simulink library "PowerFlowLib"  (R2016a)
settings: Solver=ode45  StartTime=0.0  StopTime=10.0  RelTol=1e-3
undefined symbols (not defined in the file or in its folder): Air, AirProp, C, F1, F2, Fanmap, Fld1, Fld2, Fluid, fueltankdata, HydProp, HydraulicLoad, IBFD_exc, L, LoadFluidProps, magnitude, MSSN, n_alghts, PumpProp, pwr_alghts, R_fd_exc, Rcore, Ts, VBFD_exc
libraries: PowerFlowLib x35, simulink x19, powerlib_extras x2, dspstat3 x2
(part 8 of 12)

== system PowerFlowLib/Energy & Power Systems/Electrical/Systems/Generator Bus ==
  Select : Inport
  MAIN_Gen : Inport  Port=2
  APU_Gen : Inport  Port=3
  GND_sup : Inport  Port=4
  AUX_sup : Inport  Port=5
  i_Bus : Inport  Port=6
  Compare To Constant : Subsystem  mask(Compare To Constant){relop===, const=1, LogicOutDataTypeMode=uint8, ZeroCross=on}
      mask prompts: relop "Operator:"; const "Constant value:"; LogicOutDataTypeMode "Output data type mode:"; ZeroCross "Enable zero-crossing detection"
      mask help: Determine how a signal compares to a constant.
      mask init:
      | blkName = gcb;
      | 
      | if strcmp(get_param(gcbh,'LogicOutDataTypeMode'),'boolean')
      | 	setValue = 'Boolean';
      | else
      | 	setValue = 'Specify via dialog';
      | end
      | 
      | set_param([blkName,'/Compare'],'relop',relop, ...
      | 	'LogicOutDataTypeMode', setValue, 'ZeroCross', ZeroCross);
      | 
      | str = [relop,' C']; %default
      | 
      | const_str = get_param(blkName, 'const');
      | 
      | if isempty(strfind(const_str, ' ')) && isempty(strfind(const_str, ','))
      |     % scalar or single expression
      |     if isempty(str2num(const_str))
      |         %expression
      |         str = [relop, ' ', const_str];
      |     elseif length(const) == 1
      |         str = [relop,' ',num2str(double(const))];
      |     end
      | end
      mask TypeOptions relop: == | ~= | < | <= | >= | >
      mask TypeOptions LogicOutDataTypeMode: uint8 | boolean
      mask Callback ZeroCross: sl('zeroCrossEnable', gcbh);
      mask Display: disp(str)
  Compare To Constant1 : Subsystem  mask(Compare To Constant){relop===, const=2, LogicOutDataTypeMode=uint8, ZeroCross=on}
      mask prompts: relop "Operator:"; const "Constant value:"; LogicOutDataTypeMode "Output data type mode:"; ZeroCross "Enable zero-crossing detection"
      mask help: Determine how a signal compares to a constant.
      mask init: same as PowerFlowLib/Energy & Power Systems/Electrical/Systems/Generator Bus/Compare To Constant
      mask TypeOptions relop: == | ~= | < | <= | >= | >
      mask TypeOptions LogicOutDataTypeMode: uint8 | boolean
      mask Callback ZeroCross: sl('zeroCrossEnable', gcbh);
      mask Display: disp(str)
  Compare To Constant2 : Subsystem  mask(Compare To Constant){relop===, const=3, LogicOutDataTypeMode=uint8, ZeroCross=on}
      mask prompts: relop "Operator:"; const "Constant value:"; LogicOutDataTypeMode "Output data type mode:"; ZeroCross "Enable zero-crossing detection"
      mask help: Determine how a signal compares to a constant.
      mask init: same as PowerFlowLib/Energy & Power Systems/Electrical/Systems/Generator Bus/Compare To Constant
      mask TypeOptions relop: == | ~= | < | <= | >= | >
      mask TypeOptions LogicOutDataTypeMode: uint8 | boolean
      mask Callback ZeroCross: sl('zeroCrossEnable', gcbh);
      mask Display: disp(str)
  Compare To Constant3 : Subsystem  mask(Compare To Constant){relop===, const=4, LogicOutDataTypeMode=uint8, ZeroCross=on}
      mask prompts: relop "Operator:"; const "Constant value:"; LogicOutDataTypeMode "Output data type mode:"; ZeroCross "Enable zero-crossing detection"
      mask help: Determine how a signal compares to a constant.
      mask init: same as PowerFlowLib/Energy & Power Systems/Electrical/Systems/Generator Bus/Compare To Constant
      mask TypeOptions relop: == | ~= | < | <= | >= | >
      mask TypeOptions LogicOutDataTypeMode: uint8 | boolean
      mask Callback ZeroCross: sl('zeroCrossEnable', gcbh);
      mask Display: disp(str)
  Constant : Constant  Value=[0 0 0]
  Multiport Switch : MultiPortSwitch  Inputs=4
  Switch{,1..3} (4 alike) : Switch  Criteria=u2 ~= 0  Threshold=0.5
  Vbus : Outport
  i_MAIN : Outport  Port=2
  i_APU : Outport  Port=3
  i_GND : Outport  Port=4
  i_AUX : Outport  Port=5
  wires:
  MAIN_Gen/1 -> Multiport Switch/2
  APU_Gen/1 -> Multiport Switch/3
  GND_sup/1 -> Multiport Switch/4
  AUX_sup/1 -> Multiport Switch/5
  Multiport Switch/1 -> Vbus/1
  Select/1 -> Multiport Switch/1, Compare To Constant/1(u), Compare To Constant1/1(u), Compare To Constant2/1(u), Compare To Constant3/1(u)
  Switch/1 -> i_MAIN/1
  Switch1/1 -> i_APU/1
  Switch2/1 -> i_GND/1
  Switch3/1 -> i_AUX/1
  i_Bus/1 -> Switch/1, Switch1/1, Switch2/1, Switch3/1
  Compare To Constant/1(y) -> Switch/2
  Compare To Constant1/1(y) -> Switch1/2
  Compare To Constant2/1(y) -> Switch2/2
  Compare To Constant3/1(y) -> Switch3/2
  Constant/1 -> Switch3/3, Switch2/3, Switch1/3, Switch/3

== system PowerFlowLib/Energy & Power Systems/Electrical/Systems/Inverter Phase Control ==
  Constant : Constant  Value=pi/120
  Constant5 : Constant  Value=[1 0 0]
  Demux : Demux  Outputs=3
  Mux : Mux  Inputs=3
  Scope : Scope  NumInputPorts=2
  Sum : Sum  Inputs=|++
  Trigonometric Function : Trigonometry  Operator=atan2
  Trigonometric Function1 : Trigonometry
  Trigonometric Function2 : Trigonometry  Operator=cos
  q : Outport
  wires:
  Demux/1 -> Trigonometric Function/1
  Demux/2 -> Trigonometric Function/2
  Trigonometric Function/1 -> Sum/1
  Constant/1 -> Sum/2
  Sum/1 -> Trigonometric Function1/1, Trigonometric Function2/1
  Trigonometric Function1/1 -> Mux/1
  Trigonometric Function2/1 -> Mux/2
  Demux/3 -> Mux/3
  Mux/1 -> q/1, Scope/1
  Constant5/1 -> Demux/1

== system PowerFlowLib/Energy & Power Systems/Electrical/Systems/Transformer-rectifier ==
  vqd0 : Inport
  VDC : Inport  Port=2
  Bus Creator : BusCreator  Inputs=2
  Constant : Constant  Value=0.5*pu
  Memory33 : Memory
  Transformer1 : PowerFlowLib/Energy & Power Systems/Electrical/Machines/Transformer  Rp=0.005  Rs=0.1  N1=400  N2=197
  data_sink : PowerFlowLib/Support Functions//Tools/data_sink
  rectifier1 : PowerFlowLib/Energy & Power Systems/Electrical/Converters/rectifier  L=1e-1
  iout : Outport
  iqd0 : Outport  Port=2
  wires:
  vqd0/1 -> Transformer1/1
  VDC/1 -> rectifier1/3
  Transformer1/1 -> rectifier1/1
  Constant/1 -> rectifier1/2
  Memory33/1 -> Transformer1/2
  rectifier1/2 -> Memory33/1
  Transformer1/2 -> iqd0/1
  rectifier1/1 -> iout/1, Bus Creator/1  "Rectified Current (A)"
  Bus Creator/1 -> data_sink/1

== system PowerFlowLib/Energy & Power Systems/Electrical/Systems/three-phase full-bridge inverter ==
  qabc : Inport
  VDC : Inport  Port=2
  iabc : Inport  Port=3
  Add : Sum  Inputs=+
  Product : Product  SaturateOnIntegerOverflow=on  InputSameDT=on  OutDataTypeStr=Inherit: Same as first input
  Product1 : Product  SaturateOnIntegerOverflow=on  InputSameDT=on  OutDataTypeStr=Inherit: Same as first input
  Product2 : Product  RndMeth=Zero
  Scope : Scope
  Sqrt : Sqrt  SaturateOnIntegerOverflow=on
  Sum1 : Sum  Inputs=+
  Three-Phase Full Bridge Inverter CONSTANT FREQUENCY1 : Subsystem  mask{Tr=4e-6, Tf=3e-6, Fsw=2000, VCEsat=1, Nsw=6}
      mask prompts: Tr "Rise time for switching (s)"; Tf "Fall time for switching (s)"; Fsw "PWM Frequency (Hz)"; VCEsat "VCE saturation volt (V)"; Nsw "No. switches in inverter"
  Vabc : Outport
  Idc : Outport  Port=2
  Ploss : Outport  Port=3
  wires:
  [VDC] -> Product/2
  VDC/1 -> [VDC]
  Product/1 -> Vabc/1
  iabc/1 -> Product1/1, Product2/2, Product2/1
  qabc/1 -> [qabc]
  [qabc] -> Product/1
  [qabc] -> Product1/2
  Product1/1 -> Sum1/1
  Sum1/1 -> Idc/1
  [VDC] -> Three-Phase Full Bridge Inverter CONSTANT FREQUENCY1/1(Vdc)
  Add/1 -> Sqrt/1
  Product2/1 -> Add/1
  Sqrt/1 -> Three-Phase Full Bridge Inverter CONSTANT FREQUENCY1/2(Inverter current)
  Three-Phase Full Bridge Inverter CONSTANT FREQUENCY1/1(Total Loss) -> Scope/1, Ploss/1

== system PowerFlowLib/Energy & Power Systems/Hydraulic/Hydraulic Load/Reset Timer ==
  Reset : Inport
  Clock1 : Clock
  Clock3 : Clock
  Memory : Memory
  Sum1 : Sum  Inputs=|+-  SaturateOnIntegerOverflow=on  InputSameDT=on  OutDataTypeStr=Inherit: Same as first input
  Switch2 : Switch  Threshold=1  RndMeth=Zero
  Count : Outport
  wires:
  Clock1/1 -> Sum1/1
  Clock3/1 -> Switch2/3
  Switch2/1 -> Sum1/2, Memory/1
  Sum1/1 -> Count/1
  Reset/1 -> Switch2/2
  Memory/1 -> Switch2/1

== system PowerFlowLib/Energy & Power Systems/Thermal/ECS/ACM ==
  Flow In : Inport
  "Flow In " : Inport  Port=2
  Third Stream Air : Inport  Port=3
  Bus Selector1 : BusSelector  OutputSignals=temp_K
  Compressor : Subsystem
  Expanding Turbine : Subsystem
  Mux : Mux  Inputs=3
  Power Turbine : Subsystem
  Primary Heat Exchanger : Subsystem  mask{fld1=Air, fld2=Air, Tw_init=34, C_wall=60000, flow_switch=Upstream, Tw0=50, Q0=80000, H1_0=1500, A1=2.8702, mdot1_0=3, Tin1_0=15, H2_0=1500, A2=0.10566, mdot2_0=0.91, Tin2_0=600}
      mask prompts: fld1 "Fluid Type 1"; fld2 "Fluid Type 2"; Tw_init "Initial Wall Temperature [°C]"; C_wall "Wall Heat Capacitance  [J/K]"; flow_switch "Mass Flow Rate Calculated:"; Tw0 "Wall Temperature [°C]"; Q0 "Heat Transfer Rate [W]"; H1_0 "Heat Transfer Coefficient [W/m²K]"; A1 "Heat Transfer Area [m²]"; mdot1_0 "Mass Flow Rate [kg/s]"; Tin1_0 "Fluid Inlet Temperature[°C]"; H2_0 "Heat Transfer Coefficient [W/m²K]"; A2 "Heat Transfer Area [m²]"; mdot2_0 "Mass Flow Rate [kg/s]"; Tin2_0 "Fluid Inlet Temperature[°C]"
      mask init:
      | load Fluids
      | eval(['F1 = Fluid.',get_param(gcb,'fld1'),';']);
      | eval(['F2 = Fluid.',get_param(gcb,'fld2'),';']);
      | 
      | area1 = -(mdot1_0*F1.cp/H1_0)*...
      |               log(1-Q0/(mdot1_0*F1.cp*abs(Tw0-Tin1_0)));
      | 
      | set_param(gcb,'A1',num2str(area1));          
      |           
      | area2 = -(mdot2_0*F2.cp/H2_0)*...
      |               log(1-Q0/(mdot2_0*F2.cp*abs(-Tw0+Tin2_0)));   
      |           
      | set_param(gcb,'A2',num2str(area2));
      mask TypeOptions fld1: Fuel | Water | Air
      mask TypeOptions fld2: Fuel | Water | Air
      mask TypeOptions flow_switch: Upstream | Downstream
      mask Display:
      | text(0.5,0.95,['{\bf ',fld1,'/',fld2,' HX}'],'TexMode','on','horizontalAlignment', 'center')
      | 
      | port_label('input',1,[fld1,' In'])
      | port_label('input',2,[fld2,' In'])
      | port_label('output',1,[fld1,' Out'])
      | port_label('output',2,[fld2,' Out'])
  Scope : Scope  NumInputPorts=3
  Shaft : Subsystem
  Signal Routing : Subsystem
  Terminator1 : Terminator
  Terminator2 : Terminator
  Terminator3 : Terminator
  W to HP2 : Gain  Gain=0.00134102209
  rad 2 rev : Gain  Gain=60/2/pi
  Flow Out : Outport
  RPM : Outport  Port=2
  wires:
  Mux/1 -> Shaft/1(Power In/Out [vector])
  Shaft/1(Angular Velocity [rad/s]) -> rad 2 rev/1, Expanding Turbine/2(omega_rad/s), Compressor/2(omega_rad/s)
  Compressor/2(Power [W]) -> Scope/1, Mux/1
  Expanding Turbine/1(Power [W]) -> Scope/2, Mux/2
  Power Turbine/1(Power [W]) -> W to HP2/1, Scope/3, Mux/3
  "Flow In "/1 -> Power Turbine/1(Flow In)
  Compressor/1("Flow Out ") -> Primary Heat Exchanger/1(In1)
  Expanding Turbine/2(Flow Out) -> Flow Out/1
  Signal Routing/1(Flow Out) -> Primary Heat Exchanger/2(In2)
  Power Turbine/2(Flow Out) -> Terminator1/1
  rad 2 rev/1 -> RPM/1
  Third Stream Air/1 -> Bus Selector1/1, Signal Routing/1(Flow In)
  Bus Selector1/1 -> Power Turbine/2(temp_3rd)  "<temp_K>"
  Flow In/1 -> Compressor/1(Flow In)
  Primary Heat Exchanger/1(Out1) -> Expanding Turbine/1(Flow In)
  Primary Heat Exchanger/2(Out2) -> Terminator2/1
  W to HP2/1 -> Terminator3/1

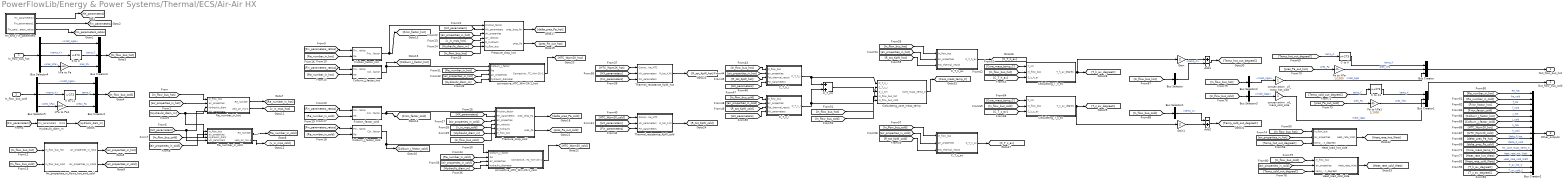
== system PowerFlowLib/Energy & Power Systems/Thermal/ECS/Air-Air HX ==
  In_flow_bus_hot : Inport
  In_flow_bus_cold : Inport  Port=2
  Add1 : Sum  Inputs=+-
  Add2 : Sum  Inputs=-+
  Air_properties_in_flows_hot_and_cold : Subsystem
  Bus Creator{,1,3..4} (4 alike) : BusCreator  Inputs=3
  Bus Creator2 : BusCreator  Inputs=15
  Bus Selector : BusSelector  OutputSignals=temp_C
  Bus Selector1 : BusSelector  OutputSignals=temp_C
  Bus Selector2 : BusSelector  OutputSignals=mdot_kgps
  Bus Selector3 : BusSelector  OutputSignals=mdot_kgps
  Bus Selector4 : BusSelector  OutputSignals=mdot_kgps,temp_K,pres_kPa
  Bus Selector5 : BusSelector  OutputSignals=mdot_kgps,temp_K,pres_kPa
  C to K : Bias  Bias=273
  C to K1 : Bias  Bias=273
  C_T_c_av : Subsystem
  C_T_c_i : Subsystem
  C_T_cm : Sum
  C_T_h_av : Subsystem
  C_T_h_i : Subsystem
  Calculating_T_c_av : Subsystem
  Calculating_T_h_av : Subsystem
  Calculating_core_mass_temp : Subsystem
  Colburn_J_factor_cold : Subsystem
  Colburn_J_factor_hot : Subsystem
  Friction_factor_cold : Subsystem
  Friction_factor_hot : Subsystem
  Gain : Gain  Gain=2
  Gain1 : Gain  Gain=2
  HX_and_Fin_paramters : Subsystem
  Heat_load_cold_side : Subsystem
  Heat_load_hot_side : Subsystem
  Hydraulic_diam_m : Subsystem
  K to C : Bias  Bias=-273
  K to C1 : Bias  Bias=-273
  Pa to kPa : Gain  Gain=1/1000
  Pa to kPa1 : Gain  Gain=1/1000
  Pressure_drop_cold : Subsystem
  Pressure_drop_hot : Subsystem
  Re_number_in_cold : Subsystem
  Re_number_in_hot : Subsystem
  Thermal_resistance_KpW_cold : Subsystem
  Thermal_resistance_KpW_hot : Subsystem
  conservation _of_mass_cold_side : Gain
  conservation _of_mass_hot_side : Gain
  convective_HTC_Wm-2K-1_cold : Subsystem
  convective_HTC_Wm-2K-1_hot : Subsystem
  kPa to Pa : Gain  Gain=1000
  kPa to Pa1 : Gain  Gain=1000
  Out_flow_bus_hot : Outport
  Out_flow_bus_cold : Outport  Port=2
  Other_outputs : Outport  Port=3
  wires:
  Heat_load_cold_side/1(Heat_rate_Watt) -> [Heat_rate_cold_Watt]
  [air_properties_in_cold] -> Heat_load_cold_side/2(air_properties)
  [In_flow_bus_cold] -> Heat_load_cold_side/1(In_flow_bus)
  [Temp_cold_out_degreeC] -> Heat_load_cold_side/3(temp_out_degreeC)
  Heat_load_hot_side/1(Heat_rate_Watt) -> [Heat_rate_hot_Watt]
  [air_properties_in_hot] -> Heat_load_hot_side/2(air_properties)
  [In_flow_bus_hot] -> Heat_load_hot_side/1(In_flow_bus)
  [Temp_hot_out_degreeC] -> Heat_load_hot_side/3(temp_out_degreeC)
  [R_tot_KpW_cold] -> C_T_c_av/3(Tot_thermal_resist)
  [air_properties_in_cold] -> C_T_c_av/2(air_properties)
  [In_flow_bus_cold] -> C_T_c_av/1(In_flow_bus)
  C_T_c_av/1(C_T_c_av) -> [C_T_c_av]
  Re_number_in_cold/2(velo_air_ms-1) -> [v_in_mps_cold]
  Bus Creator2/1 -> Other_outputs/1
  Bus Creator1/1 -> Out_flow_bus_cold/1
  Bus Creator/1 -> Out_flow_bus_hot/1
  conservation _of_mass_cold_side/1 -> Bus Creator1/3  "mdot_kgps"
  Bus Selector3/1 -> conservation _of_mass_cold_side/1  "<mdot_kgps>"
  conservation _of_mass_hot_side/1 -> Bus Creator/3  "mdot_kgps"
  Bus Selector2/1 -> conservation _of_mass_hot_side/1  "<mdot_kgps>"
  [In_flow_bus_cold] -> Bus Selector3/1
  [In_flow_bus_hot] -> Bus Selector2/1
  [pres_Pa_out_cold] -> Pa to kPa1/1  "pres_Pa"
  [Temp_cold_out_degreeC] -> C to K1/1  "temp_C"
  [pres_Pa_out_hot] -> Pa to kPa/1  "pres_Pa"
  [Temp_hot_out_degreeC] -> C to K/1  "temp_C"
  Add2/1 -> [Temp_cold_out_degreeC]
  Add1/1 -> [Temp_hot_out_degreeC]
  Bus Selector1/1 -> Add2/1  "<temp_C>"
  Gain1/1 -> Add2/2
  Bus Selector/1 -> Add1/2  "<temp_C>"
  Gain/1 -> Add1/1
  [In_flow_bus_cold] -> Bus Selector1/1
  [In_flow_bus_hot] -> Bus Selector/1
  Calculating_T_h_av/1(T_h_av_degreC) -> Gain/1, [T_h_av_degreeC]
  Calculating_T_c_av/1(T_c_av_degreC) -> Gain1/1, [T_c_av_degreeC]
  [C_T_c_av] -> Calculating_T_c_av/3(C_t_c_av)
  [In_flow_bus_cold] -> Calculating_T_c_av/2(In_flow_bus)
  [Core_mass_temp_C] -> Calculating_T_c_av/1(T_cm)
  [C_T_h_av] -> Calculating_T_h_av/3(C_t_h_av)
  C_T_h_av/1(C_T_h_av) -> [C_T_h_av]
  [In_flow_bus_hot] -> Calculating_T_h_av/2(In_flow_bus)
  [Core_mass_temp_C] -> Calculating_T_h_av/1(T_cm)
  Calculating_core_mass_temp/1(Core_mass_temp_C) -> [Core_mass_temp_C]
  [R_tot_KpW_hot] -> C_T_h_av/3(Tot_thermal_resist)
  [air_properties_in_hot] -> C_T_h_av/2(air_properties)
  [In_flow_bus_hot] -> C_T_h_av/1(In_flow_bus)
  [In_flow_bus_cold] -> Calculating_core_mass_temp/5(In_flow_bus_cold)
  [In_flow_bus_hot] -> Calculating_core_mass_temp/4(In_flow_bus_hot)
  C_T_cm/1 -> Calculating_core_mass_temp/3(C_t_cm)
  C_T_c_i/1(C_T_c_i) -> Calculating_core_mass_temp/2(C_T_c_i), C_T_cm/2
  C_T_h_i/1(C_T_h_i) -> Calculating_core_mass_temp/1(C_T_h_i), C_T_cm/1
  [HX_parameters] -> C_T_c_i/4(HX_parameters)
  [R_tot_KpW_cold] -> C_T_c_i/3(Tot_thermal_resist)
  [air_properties_in_cold] -> C_T_c_i/2(air_properties)
  [In_flow_bus_cold] -> C_T_c_i/1(In_flow_bus)
  [HX_parameters] -> C_T_h_i/4(HX_parameters)
  [R_tot_KpW_hot] -> C_T_h_i/3(Tot_thermal_resist)
  Thermal_resistance_KpW_cold/1(R_tot_K/W) -> [R_tot_KpW_cold]
  Thermal_resistance_KpW_hot/1(R_tot_K/W) -> [R_tot_KpW_hot]
  [air_properties_in_hot] -> C_T_h_i/2(air_properties)
  [In_flow_bus_hot] -> C_T_h_i/1(In_flow_bus)
  [HX_parameters] -> Thermal_resistance_KpW_cold/2(HX_parameters)
  [Fin_parameters] -> Thermal_resistance_KpW_cold/3(Fin_parameters)
  [HTC_Wpm2K_cold] -> Thermal_resistance_KpW_cold/1(Convective_HTC)
  [HX_parameters] -> Thermal_resistance_KpW_hot/2(HX_parameters)
  [Fin_parameters] -> Thermal_resistance_KpW_hot/3(Fin_parameters)
  [HTC_Wpm2K_hot] -> Thermal_resistance_KpW_hot/1(Convective_HTC)
  convective_HTC_Wm-2K-1_cold/1(Convective_HTC_Wm-2K-1) -> [HTC_Wpm2K_cold]
  convective_HTC_Wm-2K-1_hot/1(Convective_HTC_Wm-2K-1) -> [HTC_Wpm2K_hot]
  Pressure_drop_cold/2(pres_Pa) -> [pres_Pa_out_cold]
  Pressure_drop_hot/2(pres_Pa) -> [pres_Pa_out_hot]
  Pressure_drop_cold/1(pres_drop_Pa) -> [delta_pres_Pa_cold]
  Pressure_drop_hot/1(pres_drop_Pa) -> [delta_pres_Pa_hot]
  Colburn_J_factor_cold/1(Colburn_J_factor) -> convective_HTC_Wm-2K-1_cold/1(Colburn_J_factor), [Colburn_J_factor_cold]
  [Hydraulic_diam_m] -> convective_HTC_Wm-2K-1_cold/4(hydraulic_diameter)
  [air_properties_in_cold] -> convective_HTC_Wm-2K-1_cold/3(air_properties)
  [Re_number_in_cold] -> convective_HTC_Wm-2K-1_cold/2(Re)
  [Hydraulic_diam_m] -> convective_HTC_Wm-2K-1_hot/4(hydraulic_diameter)
  [air_properties_in_hot] -> convective_HTC_Wm-2K-1_hot/3(air_properties)
  [Re_number_in_hot] -> convective_HTC_Wm-2K-1_hot/2(Re)
  Colburn_J_factor_hot/1(Colburn_J_factor) -> convective_HTC_Wm-2K-1_hot/1(Colburn_J_factor), [Colburn_J_factor_hot]
  Friction_factor_cold/1(Friction_factor) -> Pressure_drop_cold/1(Friction_factor), [Fricn_factor_cold]
  [In_flow_bus_cold] -> Pressure_drop_cold/6(In_flow_bus)
  [Hydraulic_diam_m] -> Pressure_drop_cold/5(D_hydraulic)
  [v_in_mps_cold] -> Pressure_drop_cold/4(air_velocity)
  [air_properties_in_cold] -> Pressure_drop_cold/3(air_properties)
  [HX_parameters] -> Pressure_drop_cold/2(HX_parameters)
  [In_flow_bus_hot] -> Pressure_drop_hot/6(In_flow_bus)
  Friction_factor_hot/1(Friction_factor) -> Pressure_drop_hot/1(Friction_factor), [Fricn_factor_hot]
  [Hydraulic_diam_m] -> Pressure_drop_hot/5(D_hydraulic)
  [v_in_mps_hot] -> Pressure_drop_hot/4(air_velocity)
  [air_properties_in_hot] -> Pressure_drop_hot/3(air_properties)
  [HX_parameters] -> Pressure_drop_hot/2(HX_parameters)
  Re_number_in_hot/2(velo_air_ms-1) -> [v_in_mps_hot]
  [Re_number_in_cold] -> Colburn_J_factor_cold/2(Re)
  [Fin_parameters_ratios] -> Colburn_J_factor_cold/1(Fin_prameter_ratios)
  [Re_number_in_cold] -> Friction_factor_cold/2(Re)
  [Fin_parameters_ratios] -> Friction_factor_cold/1(Fin_prameter_ratios)
  [Re_number_in_hot] -> Colburn_J_factor_hot/2(Re)
  [Fin_parameters_ratios] -> Colburn_J_factor_hot/1(Fin_prameter_ratios)
  [Re_number_in_hot] -> Friction_factor_hot/2(Re)
  [Fin_parameters_ratios] -> Friction_factor_hot/1(Fin_prameter_ratios)
  HX_and_Fin_paramters/3(Fin_parameters_ratios) -> [Fin_parameters_ratios]
  [air_properties_in_cold] -> Re_number_in_cold/2(air_properties)
  [In_flow_bus_cold] -> Re_number_in_cold/1(In_flow_bus)
  [HX_parameters] -> Re_number_in_cold/4(HX_paramters), Re_number_in_hot/4(HX_paramters)
  [Hydraulic_diam_m] -> Re_number_in_cold/3(Hydraulic_diam), Re_number_in_hot/3(Hydraulic_diam)
  [air_properties_in_hot] -> Re_number_in_hot/2(air_properties)
  [In_flow_bus_hot] -> Re_number_in_hot/1(In_flow_bus)
  [In_flow_bus_cold] -> Air_properties_in_flows_hot_and_cold/2(In_flow_bus_cold)
  [In_flow_bus_hot] -> Air_properties_in_flows_hot_and_cold/1(In_flow_bus_hot)
  Air_properties_in_flows_hot_and_cold/2(air_properties_in_cold1) -> [air_properties_in_cold]
  Air_properties_in_flows_hot_and_cold/1(air_properties_in_hot1) -> [air_properties_in_hot]
  HX_and_Fin_paramters/2(Fin_parameters1) -> [Fin_parameters]
  HX_and_Fin_paramters/1(HX_parameters2) -> [HX_parameters]
  Re_number_in_cold/1(Re_number) -> [Re_number_in_cold]
  Re_number_in_hot/1(Re_number) -> [Re_number_in_hot]
  Hydraulic_diam_m/1(Out1) -> [Hydraulic_diam_m]
  [Fin_parameters] -> Hydraulic_diam_m/1(Fin_parameters)
  C to K/1 -> Bus Creator/1  "temp_K"
  Pa to kPa/1 -> Bus Creator/2  "pres_kPa"
  C to K1/1 -> Bus Creator1/1  "temp_K"
  Pa to kPa1/1 -> Bus Creator1/2  "pres_kPa"
  [Heat_rate_cold_Watt] -> Bus Creator2/13  "Heat_rate_cold_Watt"
  [Heat_rate_hot_Watt] -> Bus Creator2/12  "Heat_rate_hot_Watt"
  [Core_mass_temp_C] -> Bus Creator2/11  "HX_core_mass_temp_C"
  [Fricn_factor_hot] -> Bus Creator2/3  "f_hot"
  [Fricn_factor_cold] -> Bus Creator2/4  "f_cold"
  [Colburn_J_factor_hot] -> Bus Creator2/5  "J_hot"
  [Colburn_J_factor_cold] -> Bus Creator2/6  "J_cold"
  [HTC_Wpm2K_hot] -> Bus Creator2/7  "h_hot"
  [HTC_Wpm2K_cold] -> Bus Creator2/8  "h_cold"
  [delta_pres_Pa_hot] -> Bus Creator2/9  "Delta_P_hot"
  [delta_pres_Pa_cold] -> Bus Creator2/10  "Delta_P_cold"
  [Re_number_in_hot] -> Bus Creator2/1  "Re_hot"
  [Re_number_in_cold] -> Bus Creator2/2  "Re_cold"
  In_flow_bus_hot/1 -> Bus Selector4/1
  Bus Selector4/1 -> Bus Creator3/1  "<mdot_kgps>"
  Bus Selector4/2 -> K to C/1  "<temp_K>"
  Bus Selector4/3 -> kPa to Pa/1  "<pres_kPa>"
  K to C/1 -> Bus Creator3/2  "temp_C"
  Bus Creator3/1 -> [In_flow_bus_hot]
  kPa to Pa/1 -> Bus Creator3/3  "pres_Pa"
  Bus Selector5/1 -> Bus Creator4/1  "<mdot_kgps>"
  Bus Selector5/2 -> K to C1/1  "<temp_K>"
  Bus Selector5/3 -> kPa to Pa1/1  "<pres_kPa>"
  K to C1/1 -> Bus Creator4/2  "temp_C"
  kPa to Pa1/1 -> Bus Creator4/3  "press_Pa"
  Bus Creator4/1 -> [In_flow_bus_cold]
  [T_h_av_degreeC] -> Bus Creator2/14  "T_av_hot_C"
  [T_c_av_degreeC] -> Bus Creator2/15  "T_av_cold_C"
  In_flow_bus_cold/1 -> Bus Selector5/1

== system PowerFlowLib/Energy & Power Systems/Thermal/ECS/Cabin Zone ==
  note: Saturation added to
      | remove division by Zero
  Supply Air Flow In : Inport
  Amb Temp [K] : Inport  Port=2
  Mach_no : Inport  Port=3
  Thermal Load : Inport  Port=4
  Air Properties : Subsystem
  Bias : Bias  Bias=-273.15
  Bus Creator1 : BusCreator  Inputs=4
  Bus Creator2 : BusCreator  Inputs=2
  Bus Creator3 : BusCreator  Inputs=3
  Bus Creator4 : BusCreator  Inputs=3
  Bus Selector1 : BusSelector  OutputSignals=Cp_ra
  Bus Selector2 : BusSelector  OutputSignals=temp_K,mdot_kgps
  Bus Selector3 : BusSelector  OutputSignals=m_dot_ra
  C to K : Bias  Bias=273.15
  C to K1 : Bias  Bias=273.15
  Cabin Pressurization : Subsystem
  Cabin Temperature : Subsystem
  Cabin_parameters : Subsystem
  Gain : Gain
  Saturation : Saturate  UpperLimit=inf  LowerLimit=eps
  Terminator : Terminator
  calc_recirc_temp_ from_cab_temp : Sum
  data_sink : PowerFlowLib/Support Functions//Tools/data_sink
  m_dot_sa_required1 : Subsystem
  t_sa_term : Product  Inputs=*//
  Cabin Conditions : Outport
  Return Air  Conditions : Outport  Port=2
  wires:
  Saturation/1 -> t_sa_term/3
  calc_recirc_temp_ from_cab_temp/1 -> C to K1/1
  t_sa_term/1 -> calc_recirc_temp_ from_cab_temp/2
  [temp_cabin_C] -> calc_recirc_temp_ from_cab_temp/1
  Bus Selector3/1 -> Saturation/1, Gain/1  "<m_dot_ra>"
  Bus Selector1/1 -> t_sa_term/2  "<Cp_ra>"
  [Masses_cabin] -> Bus Selector3/1
  C to K1/1 -> Bus Creator3/1  "temp_K"
  Thermal Load/1 -> t_sa_term/1, Bus Creator4/3  "Thermal_Load"
  Mach_no/1 -> Cabin Temperature/6(Mach #)
  Amb Temp [K]/1 -> Cabin Temperature/5(Amb Temp [K])
  Supply Air Flow In/1 -> Bus Selector2/1, Air Properties/1(Supply Air)
  [temp_cabin_C] -> Cabin Pressurization/2(Cabin Temp. [C])
  Cabin Temperature/1(Cabin Temp. [C]) -> [temp_cabin_C], C to K/1  "temp_cabin_C"
  C to K/1 -> Bus Creator2/2, Bus Creator4/1  "temp_K"
  Bias/1 -> Cabin Temperature/1(Sup. Air Temp [C])
  m_dot_sa_required1/1(mdot SA Req.) -> Terminator/1
  Air Properties/3(Exhaust_AirProp) -> Bus Creator1/4
  Air Properties/2(Recirc_AirProp) -> Bus Selector1/1, Bus Creator1/3
  Air Properties/1(Supply_AirProp) -> m_dot_sa_required1/2(Sup. Air Prop.), Bus Creator1/2
  Bus Selector2/1 -> Bias/1  "<temp_K>"
  Air Properties/4(Cabin_AirProp) -> Cabin Pressurization/3(Cabin Prop.), Bus Creator1/1
  Cabin Pressurization/1(Cabin mdot & mass) -> [Masses_cabin], Cabin Temperature/2(Cabin mdot & mass)
  Cabin_parameters/1(Cabin Parameters) -> m_dot_sa_required1/1(Cabin Param.), Cabin Pressurization/4(Cabin Param.), Cabin Temperature/3(Cabin Param.)
  Bus Selector2/2 -> Cabin Pressurization/1(Sup. Air mdot)  "<mdot_kgps>"
  Bus Creator1/1 -> Cabin Temperature/4(Air Props.)
  Cabin Pressurization/2(Cabin Pres.) -> Bus Creator2/1, Bus Creator3/2, Bus Creator4/2  "pres_kPa"
  Bus Creator2/1 -> Cabin Conditions/1
  Bus Creator3/1 -> Return Air  Conditions/1
  Gain/1 -> Bus Creator3/3  "mdot_kgps"
  Bus Creator4/1 -> data_sink/1

== system PowerFlowLib/Energy & Power Systems/Thermal/ECS/Cargo bay ==
  note: Upper limit
      | to cargo temp.,
      | T_limit
  Return Air  Conditions : Inport
  "Thermal Loads, Q" : Inport  Port=2
  Flow from Right Pack : Inport  Port=3
  Add : Sum  Inputs=+++
  Add1 : Sum
  Bias : Bias  Bias=0.001
  Bus Creator : BusCreator  Inputs=3
  Bus Selector1 : BusSelector  OutputSignals=temp_K,mdot_kgps
  Bus Selector2 : BusSelector  OutputSignals=mdot_kgps,temp_K,pres_kPa
  Constant1 : Constant  Value=T_cargo_K
  Gain : Gain
  M_ra  x T_ra : Product
  M_right  x T_right : Product
  PID Controller1 : simulink/Continuous/PID Controller  Controller=PID  TimeDomain=Continuous-time  SampleTime=1  IntegratorMethod=Forward Euler  FilterMethod=Forward Euler  Form=Parallel  P=0.01  I=.01  D=0.01  N=100  InitialConditionSource=internal  InitialConditionForIntegrator=0  InitialConditionForFilter=0  ExternalReset=none  LimitOutput=on  UpperSaturationLimit=0.5  LowerSaturationLimit=.01  LinearizeAsGain=off  AntiWindupMode=none  Kb=1  TrackingMode=off  Kt=1  PParamMin=[]  PParamMax=[]  IParamMin=[]  IParamMax=[]  DParamMin=[]  DParamMax=[]  NParamMin=[]  NParamMax=[]  KbParamMin=[]  KbParamMax=[]  KtParamMin=[]  KtParamMax=[]  POutMin=[]  POutMax=[]  IOutMin=[]  IOutMax=[]  DOutMin=[]  DOutMax=[]  NOutMin=[]  NOutMax=[]  KbOutMin=[]  KbOutMax=[]  KtOutMin=[]  KtOutMax=[]  IntegratorOutMin=[]  IntegratorOutMax=[]  FilterOutMin=[]  FilterOutMax=[]  SumOutMin=[]  SumOutMax=[]  SumI1OutMin=[]  SumI1OutMax=[]  SumI2OutMin=[]  SumI2OutMax=[]  SumI3OutMin=[]  SumI3OutMax=[]  SumDOutMin=[]  SumDOutMax=[]  SaturationOutMin=[]  SaturationOutMax=[]  IntegratorContinuousStateAttributes=''  IntegratorStateMustResolveToSignalObject=off  IntegratorRTWStateStorageClass=Auto  FilterContinuousStateAttributes=''  FilterStateMustResolveToSignalObject=off  FilterRTWStateStorageClass=Auto
  Q/Cp : Product  Inputs=*/
  "Specific heat, Cp" : Constant  Value=1005
  Sum1 : Sum  Inputs=-+|
  T_out : Product  Inputs=*/
  data_sink : PowerFlowLib/Support Functions//Tools/data_sink
  Flow Distributor : Outport
  From cargo to fan : Outport  Port=2
  wires:
  Bias/1 -> Bus Creator/2, T_out/2  "mdot_kgps"
  M_ra  x T_ra/1 -> Add/3
  T_out/1 -> Sum1/2, Bus Creator/1  "temp_K"
  Bus Selector2/3 -> Gain/1  "<pres_kPa>"
  Bus Creator/1 -> data_sink/1, From cargo to fan/1
  Add/1 -> T_out/1
  Q/Cp/1 -> Add/2
  "Specific heat, Cp"/1 -> Q/Cp/2
  "Thermal Loads, Q"/1 -> Q/Cp/1
  Bus Selector2/2 -> M_ra  x T_ra/2  "<temp_K>"
  Bus Selector2/1 -> M_ra  x T_ra/1, Add1/2  "<mdot_kgps>"
  Add1/1 -> Bias/1  "mdot_kgps"
  M_right  x T_right/1 -> Add/1
  Bus Selector1/2 -> M_right  x T_right/2, Add1/1  "<mdot_kgps>"
  Bus Selector1/1 -> M_right  x T_right/1  "<temp_K>"
  Flow from Right Pack/1 -> Bus Selector1/1
  Sum1/1 -> PID Controller1/1
  Return Air  Conditions/1 -> Bus Selector2/1
  Constant1/1 -> Sum1/1
  PID Controller1/1 -> Flow Distributor/1  "Increase flow rate from the right pack"
  Gain/1 -> Bus Creator/3  "pres_kPa"

== system PowerFlowLib/Energy & Power Systems/Thermal/ECS/Compressor ==
  note: eff
  note: N
  note: Flow
  In2 : Inport
  In4 : Inport  Port=2
  Add : Sum
  Bias : Bias  Bias=-1
  Bus Creator1 : BusCreator  Inputs=3
  Bus Selector : BusSelector  OutputSignals=pres_kPa
  Bus Selector1 : BusSelector  OutputSignals=mdot_kgps
  Bus Selector2 : BusSelector  OutputSignals=temp_K
  Cp(P,T)1 : Lookup_n-D  BreakpointsForDimension1=AirProp.P  BreakpointsForDimension2=AirProp.T  BreakpointsForDimension3=[1]  Table=AirProp.Cp_pt  RndMeth=Simplest  InputSameDT=on
  Divide1 : Product  Inputs=/**
  Divide2 : Product  Inputs=***
  Divide3 : Product  Inputs=**
  Divide4 : Product  Inputs=/*
  Divide5 : Product  Inputs=/**
  Gain1 : Gain  Gain=1000
  K to R : Gain  Gain=1.8
  Math Function : Math  Operator=pow  SaturateOnIntegerOverflow=on
  Pressure_ratio : Lookup_n-D  BreakpointsForDimension1=[20,25,30,35,40,45,50,55,60,65,70,75,80,85,90]  BreakpointsForDimension2=[1097,1316,1536,1756,1975,2195,2414]  Table=reshape([1.22,1.202,1.18,1.145,1.05,1,1,1,1,1,1,1,1,1,1,1.325,1.31,1.3,1.275,1.22,1.16,1,1,1,1,1,1,1,1,1,1.49,1.485,1.475,1.45,1.41,1.38,1.3,1.15,1,1,1,1,1,1,1,1.65,1.65,1.63,1.628,1.61,1.598,1.55,1.5,1.4,1.1,1,1,1,1,1,1.885,1.87,1.87,1.86,1.83,1.82,1.8,1.76,1.7,1.62,1.5,1,1,1,1,2.15,2.15,2.15,2.14,2.12,2.05,2.085,2.05,2.01,1.98,1.902,1.8,1,1,1,2.45,2.44,2.43,2.42,2.41,2.405,2.4,2.39,2.365,2.32,2.28,2.2,2.14,2.02,1.7],15,7)  RndMeth=Simplest  InputSameDT=on
  Reciprocal Sqrt : Sqrt  SaturateOnIntegerOverflow=on
  Table1 : Lookup_n-D  BreakpointsForDimension1=[20,25,30,35,40,45,50,55,60,65,70,75,80,85,90]  BreakpointsForDimension2=[1097,1316,1536,1756,1975,2195,2414]  Table=reshape([0.84396,0.83224,0.7928,0.70795,0.33,0.16,0.16,0.16,0.16,0.16,0.16,0.16,0.16,0.16,0.16,0.8265,0.8272,0.823,0.8075,0.709,0.5437,0.0850000000000002,0.0850000000000002,0.0850000000000002,0.0850000000000002,0.0850000000000002,0.0850000000000002,0.0850000000000002,0.0850000000000002,0.0850000000000002,0.6962,0.716699999999999,0.753,0.8086,0.8094,0.777,0.672,0.3705,0.0690000000000002,0.0690000000000002,0.0690000000000002,0.0690000000000002,0.0690000000000002,0.0690000000000002,0.0690000000000002,0.803,0.803,0.8122,0.81312,0.82042,0.822052,0.8045,0.755,0.654,0.192,0.0480000000000002,0.0480000000000002,0.0480000000000002,0.0480000000000002,0.0480000000000002,0.79155,0.8025,0.8025,0.806,0.81335,0.8144,0.8165,0.811,0.7775,0.7328,0.628,0.0080000000000004,0.0080000000000004,0.0080000000000004,0.0080000000000004,0.802,0.802,0.802,0.802,0.802,0.8112,0.80584,0.8112,0.81728,0.80648,0.77466,0.723,0.00180000000000019,0.00180000000000019,0.00180000000000019,0.81,0.81,0.81,0.81,0.81,0.81,0.81,0.81,0.81,0.81,0.8068,0.7888,0.766,0.72408,0.54796],15,7)  RndMeth=Simplest  InputSameDT=on
  "m and P " : Gain  Gain=900
  poly index : Constant  Value=(1.4-1)/1.4
  Out1 : Outport
  Power_out : Outport  Port=2
  wires:
  Table1/1 -> Divide1/1
  "m and P "/1 -> Table1/1, Pressure_ratio/1
  Divide5/1 -> "m and P "/1
  Divide4/1 -> Table1/2, Pressure_ratio/2
  In4/1 -> Divide4/2
  K to R/1 -> Reciprocal Sqrt/1
  Bus Creator1/1 -> Out1/1
  Add/1 -> Bus Creator1/3  "temp_K"
  Divide3/1 -> Bus Creator1/1, Cp(P,T)1/1  "pres_kPa"
  Bus Selector/1 -> Divide5/1, Divide3/1  "<pres_kPa>"
  Divide2/1 -> Power_out/1
  Divide1/1 -> Add/1, Divide2/3, Cp(P,T)1/2
  Bias/1 -> Divide1/2
  Math Function/1 -> Bias/1
  poly index/1 -> Math Function/2
  Pressure_ratio/1 -> Divide3/2, Math Function/1
  Bus Selector1/1 -> Divide5/2, Bus Creator1/2, Divide2/1  "<mdot_kgps>"
  Reciprocal Sqrt/1 -> Divide5/3, Divide4/1
  Bus Selector2/1 -> K to R/1, Add/2, Divide1/3  "<temp_K>"
  In2/1 -> Bus Selector2/1, Bus Selector1/1, Bus Selector/1
  Cp(P,T)1/1 -> Gain1/1
  Gain1/1 -> Divide2/2

== system PowerFlowLib/Energy & Power Systems/Thermal/ECS/Fan ==
  Flow In : Inport
  Air Properties : Subsystem
  Bias : Bias  Bias=-273
  Bias1 : Bias  Bias=273
  Bus Creator{2,4..6} (4 alike) : BusCreator  Inputs=3
  Bus Selector : BusSelector  OutputSignals=Rho_in_kgpm3
  Bus Selector1 : BusSelector  OutputSignals=mdot_kgps
  Bus Selector2 : BusSelector  OutputSignals=mdot_kgps,temp_C,press_Pa
  Bus Selector3 : BusSelector  OutputSignals=temp_K,pres_kPa,mdot_kgps
  Calculating_vol_flow_rate : Product  Inputs=*/
  Constant : Constant  Value=N_fan
  Gain : Gain  Gain=1000
  Gain1 : Gain  Gain=1/1000
  Gain2 : Gain
  Gain3 : Gain
  Gain4 : Gain  Gain=1/1000
  Performance_curves_1725 rpm : Subsystem  TreatAsAtomicUnit=on
  m3ps_to_cfm : Gain  Gain=2118.88
  Flow Out : Outport
  Fan Data : Outport  Port=2
  wires:
  Constant/1 -> [Fan_speed_rpm]
  Bus Selector3/1 -> Bias/1  "<temp_K>"
  Gain4/1 -> Bus Creator5/2  "power_kW"
  Performance_curves_1725 rpm/1(Power_required_W) -> Gain4/1  "power_W"
  [Fan_speed_rpm] -> Bus Creator5/1  "fan_speed_rpm"
  Performance_curves_1725 rpm/2(fan_efficiency) -> Bus Creator5/3  "fan_efficiency"
  Performance_curves_1725 rpm/5(mass_kgps) -> Bus Creator4/3
  Performance_curves_1725 rpm/4(Temp_out_C) -> Bus Creator4/2
  Performance_curves_1725 rpm/3(Pressure_out_Pa) -> Bus Creator4/1
  Bus Creator4/1 -> Bus Selector2/1
  Bus Creator6/1 -> Flow Out/1
  Bus Creator5/1 -> Fan Data/1
  Bus Selector2/3 -> Gain1/1  "<press_Pa>"
  Bus Selector2/2 -> Bias1/1  "<temp_C>"
  Bus Selector2/1 -> Gain3/1  "<mdot_kgps>"
  Bias1/1 -> Bus Creator6/2  "temp_K"
  Gain1/1 -> Bus Creator6/3  "pres_kPa"
  Gain3/1 -> Bus Creator6/1  "mdot_kgps"
  [FlowIn] -> Performance_curves_1725 rpm/2(in_flow_bus)
  [Vol_flow_rate] -> Performance_curves_1725 rpm/1(Vol_flow_rate_cfm_in)
  [AirProp] -> Performance_curves_1725 rpm/3(Air_properties_at_inlet)
  m3ps_to_cfm/1 -> [Vol_flow_rate]
  Calculating_vol_flow_rate/1 -> m3ps_to_cfm/1
  Bus Selector1/1 -> Calculating_vol_flow_rate/1  "<mdot_kgps>"
  [FlowIn] -> Bus Selector1/1
  Bus Selector/1 -> Calculating_vol_flow_rate/2  "<Rho_in_kgpm3>"
  Air Properties/1(AirProp) -> [AirProp], Bus Selector/1
  Bus Creator2/1 -> [FlowIn]
  Flow In/1 -> Air Properties/1(Flow In), Bus Selector3/1
  Bias/1 -> Bus Creator2/1  "temp_C"
  Gain/1 -> Bus Creator2/2  "pres_Pa"
  Gain2/1 -> Bus Creator2/3  "mdot_kgps"
  Bus Selector3/2 -> Gain/1  "<pres_kPa>"
  Bus Selector3/3 -> Gain2/1  "<mdot_kgps>"

== system PowerFlowLib/Energy & Power Systems/Thermal/ECS/T_35_valve ==
  In1 : Inport
  In2 : Inport  Port=2
  Bus Creator1 : BusCreator  Inputs=3
  Bus Creator2 : BusCreator  Inputs=3
  Bus Selector1 : BusSelector  OutputSignals=temp_K,mdot_kgps,pres_kPa
  Bus Selector3 : BusSelector  OutputSignals=temp_K,mdot_kgps,pres_kPa
  Constant2 : Constant  Value=0
  Memoy1 : Memory
  Scope : Scope
  Subtract2 : Sum  Inputs=+-
  Subtract3 : Sum  Inputs=+-
  Subtract4 : Sum  Inputs=+-
  Switch2 : Switch
  Switch3 : Switch
  T_35F : Constant  Value=T_35
  Terminator : Terminator
  delta_m =m_c*(T_35-Tt)/(Tc-Tt) : Product  Inputs=/**
  Out2 : Outport
  Out1 : Outport  Port=2
  wires:
  T_35F/1 -> Subtract2/1, Switch3/1
  Bus Selector3/1 -> Subtract3/2, Subtract2/2, Switch3/3  "<temp_K>"
  Subtract2/1 -> delta_m =m_c*(T_35-Tt)/(Tc-Tt)/3
  Bus Selector1/2 -> delta_m =m_c*(T_35-Tt)/(Tc-Tt)/2, Subtract4/1, Bus Creator2/2  "<mdot_kgps>"
  Bus Selector1/1 -> Subtract3/1, Bus Creator1/1  "<temp_K>"
  Subtract3/1 -> delta_m =m_c*(T_35-Tt)/(Tc-Tt)/1
  delta_m =m_c*(T_35-Tt)/(Tc-Tt)/1 -> Switch2/2, Switch2/1, Switch3/2  "delta_m"
  Constant2/1 -> Switch2/3
  Switch2/1 -> Memoy1/1
  Bus Selector1/3 -> Bus Creator1/2  "<pres_kPa>"
  Memoy1/1 -> Subtract4/2, Scope/1
  Subtract4/1 -> Bus Creator1/3  "mdot_kgps"
  Bus Creator1/1 -> Out1/1
  Switch3/1 -> Bus Creator2/1  "temp_K"
  Bus Selector3/3 -> Bus Creator2/3  "<pres_kPa>"
  Bus Selector3/2 -> Terminator/1  "<mdot_kgps>"
  Bus Creator2/1 -> Out2/1
  In1/1 -> Bus Selector1/1
  In2/1 -> Bus Selector3/1

== system PowerFlowLib/Energy & Power Systems/Thermal/ECS/Turbine ==
  note: Pt
  Flow : Inport
  W_compressor : Inport  Port=2
  Add : Sum  Inputs=+-
  Add1 : Sum  Inputs=-+
  Bias : Bias  Bias=-1
  Bus Creator : BusCreator  Inputs=3
  Bus Selector : BusSelector  OutputSignals=pres_kPa
  Bus Selector1 : BusSelector  OutputSignals=mdot_kgps
  Bus Selector2 : BusSelector  OutputSignals=temp_K
  Cp(P,T)1 : Lookup_n-D  BreakpointsForDimension1=AirProp.P  BreakpointsForDimension2=AirProp.T  BreakpointsForDimension3=[1]  Table=AirProp.Cp_pt  RndMeth=Simplest  InputSameDT=on
  Divide : Product  Inputs=/*
  Divide3 : Product  Inputs=***
  Divide4 : Product  Inputs=***
  Divide5 : Product  Inputs=/*
  Gain : Gain  Gain=-1
  Gain1 : Gain  Gain=1000
  Inertia : Constant  Value=inertia
  Integrator : Integrator  InitialCondition=1600000000
  Math Function : Math  Operator=pow  SaturateOnIntegerOverflow=on
  Reciprocal Sqrt : Sqrt  SaturateOnIntegerOverflow=on
  poly index : Constant  Value=(1.4-1)/1.4
  turbine efficiency : Constant  Value=n_t
  urbine Exit pressure : Constant  Value=press_Turbine_exit
  Flow_out : Outport
  N : Outport  Port=2
  W_turbine : Outport  Port=3
  wires:
  Bus Creator/1 -> Flow_out/1
  Gain/1 -> Divide3/2
  turbine efficiency/1 -> Divide3/3
  urbine Exit pressure/1 -> Divide/2, Bus Creator/3, Cp(P,T)1/2  "pres_kPa"
  Reciprocal Sqrt/1 -> N/1
  W_compressor/1 -> Add1/1
  Flow/1 -> Bus Selector2/1, Bus Selector1/1, Bus Selector/1
  Bus Selector/1 -> Divide/1  "<pres_kPa>"
  Divide/1 -> Math Function/1
  poly index/1 -> Math Function/2
  Math Function/1 -> Bias/1
  Bias/1 -> Gain/1
  Bus Selector2/1 -> Divide3/1, Add/1, Cp(P,T)1/1  "<temp_K>"
  Divide3/1 -> Divide4/3, Add/2
  Cp(P,T)1/1 -> Gain1/1
  Bus Selector1/1 -> Divide4/1, Bus Creator/1  "<mdot_kgps>"
  Divide4/1 -> W_turbine/1, Add1/2
  Add1/1 -> Divide5/2
  Inertia/1 -> Divide5/1
  Divide5/1 -> Integrator/1
  Integrator/1 -> Reciprocal Sqrt/1
  Add/1 -> Bus Creator/2  "temp_K"
  Gain1/1 -> Divide4/2

== system PowerFlowLib/Energy & Power Systems/Thermal/ECS/n-intlet Mixing Junction ==
  Inlet#1 : Inport
  Inlet#2 : Inport  Port=2
  Inlet#3 : Inport  Port=3
  Bias1 : Bias  Bias=-273
  Bias2 : Bias  Bias=273
  Bus Creator3 : BusCreator  Inputs=3
  BusSel#1 : BusSelector  OutputSignals=pres_kPa,temp_K,mdot_kgps
  BusSel#2 : BusSelector  OutputSignals=pres_kPa,temp_K,mdot_kgps
  BusSel#3 : BusSelector  OutputSignals=pres_kPa,temp_K,mdot_kgps
  Cp(P,T)2 : Lookup_n-D  BreakpointsForDimension1=AirProp.P  BreakpointsForDimension2=AirProp.T  BreakpointsForDimension3=[1]  Table=AirProp.Cp_pt  RndMeth=Simplest  InputSameDT=on
  Divide : Product  Inputs=***
  Divide1 : Product  Inputs=*/
  Divide2 : Product  Inputs=*/
  Divide3 : Product  Inputs=*//
  Gain1 : Gain  Gain=1000
  Sum of Elements{1..4} (4 alike) : Sum  Inputs=+
  Width : Width
  Width1 : Width
  mdot_vector : Concatenate  NumInputs=3
  pres_vector : Concatenate  NumInputs=3
  temp_vector : Concatenate  NumInputs=3
  Flow Out : Outport
  wires:
  Bias2/1 -> Bus Creator3/2  "temp_K"
  Bus Creator3/1 -> Flow Out/1
  temp_vector/1 -> Bias1/1  "temp_K"
  pres_vector/1 -> Cp(P,T)2/1, Sum of Elements4/1, Width1/1  "pres_kPa"
  Cp(P,T)2/1 -> Gain1/1  "Cp"
  mdot_vector/1 -> Sum of Elements1/1, Divide/3  "mdot"
  Sum of Elements1/1 -> Divide3/3, Bus Creator3/3  "mdot_kgps"
  Sum of Elements2/1 -> Divide2/1
  Width/1 -> Divide2/2
  Divide/1 -> Sum of Elements3/1
  Sum of Elements3/1 -> Divide3/1
  Divide2/1 -> Divide3/2
  Bias1/1 -> Divide/2, Cp(P,T)2/2
  Divide3/1 -> Bias2/1  "temp_C"
  Inlet#1/1 -> BusSel#1/1
  BusSel#1/1 -> pres_vector/1  "<pres_kPa>"
  BusSel#1/2 -> temp_vector/1  "<temp_K>"
  BusSel#1/3 -> mdot_vector/1  "<mdot_kgps>"
  Inlet#2/1 -> BusSel#2/1
  BusSel#2/1 -> pres_vector/2  "<pres_kPa>"
  BusSel#2/2 -> temp_vector/2  "<temp_K>"
  BusSel#2/3 -> mdot_vector/2  "<mdot_kgps>"
  Inlet#3/1 -> BusSel#3/1
  BusSel#3/1 -> pres_vector/3  "<pres_kPa>"
  BusSel#3/2 -> temp_vector/3  "<temp_K>"
  BusSel#3/3 -> mdot_vector/3  "<mdot_kgps>"
  Divide1/1 -> Bus Creator3/1  "pres_kPa"
  Sum of Elements4/1 -> Divide1/1
  Width1/1 -> Divide1/2
  Gain1/1 -> Sum of Elements2/1, Width/1, Divide/1

== system PowerFlowLib/Energy & Power Systems/Thermal/Fuel & Oil/Cold Plate ==
  Q : Inport
  In : Inport  Port=2
  Add : Sum  Inputs=+-
  Add1 : Sum  Inputs=-+
  Add2 : Sum
  Add3 : Sum  Inputs=-+
  Bias : Bias  Bias=eps
  Bus Creator : BusCreator  Inputs=3
  Bus Creator1 : BusCreator  Inputs=3
  Bus Selector : BusSelector  OutputSignals=mdot_kgps,temp_K,pres_kPa
  Cw : Constant  Value=C_wall
  Divide : Product  Inputs=*/
  Divide1 : Product  Inputs=**
  Divide2 : Product  Inputs=**
  Divide3 : Product  Inputs=**
  Divide4 : Product  Inputs=/**
  Gain : Gain  Gain=-1
  H_As1 : Constant  Value=4/5
  H_As4 : Constant  Value=(H0/mdot0^(4/5))*A
  Math Function : Math  SaturateOnIntegerOverflow=on
  Math Function3 : Math  Operator=pow  SaturateOnIntegerOverflow=on
  Tw : Integrator  InitialCondition=Tw_init
  cp : Constant  Value=Fluid.cp
  data_sink : PowerFlowLib/Support Functions//Tools/data_sink
  Out : Outport
  wires:
  Bias/1 -> Divide4/1
  Divide/1 -> Tw/1
  Cw/1 -> Divide/2
  Add/1 -> Divide/1
  cp/1 -> Divide1/1
  Add2/1 -> Bus Creator1/2, [T_out]  "T_out"
  Divide2/1 -> Add/2  "Q"
  Tw/1 -> Bus Creator1/1, Add2/1, Add3/1  "T_wall"
  Divide3/1 -> Add2/2
  Add3/1 -> Divide3/1
  Bus Creator/1 -> Out/1
  [m_dot] -> Bus Creator/1  "mdot_kgps"
  Q/1 -> [Q_Load]
  [Q_Load] -> Add/1
  Bus Selector/2 -> [T_in]  "<temp_K>"
  [T_in] -> Add1/1
  [T_out] -> Add1/2
  [T_out] -> Bus Creator/2  "temp_K"
  [T_in] -> Add3/2
  Math Function/1 -> Divide3/2
  Add1/1 -> Divide2/1
  Divide1/1 -> Divide2/2, Bias/1
  Divide4/1 -> Gain/1
  H_As4/1 -> Divide4/2
  Gain/1 -> Math Function/1
  Bus Selector/1 -> [m_dot]  "<mdot_kgps>"
  In/1 -> Bus Selector/1
  [m_dot] -> Math Function3/1, Divide1/2
  H_As1/1 -> Math Function3/2
  Math Function3/1 -> Divide4/3
  Bus Creator1/1 -> data_sink/1
  [Q_Load] -> Bus Creator1/3  "Q_load"
  Bus Selector/3 -> [pres_in]  "<pres_kPa>"
  [pres_in] -> Bus Creator/3  "pres_kPa"

== system PowerFlowLib/Energy & Power Systems/Thermal/Fuel & Oil/Flow Junction ==
  mdot Out : Inport
  Flow In 1 : Inport  Port=2
  Flow In 2 : Inport  Port=3
  Flow In 3 : Inport  Port=4
  Bus Creator : BusCreator  Inputs=4
  Bus Selector : BusSelector  OutputSignals=H_kJpkg
  Bus Selector1 : BusSelector  OutputSignals=H_kJpkg
  Bus Selector2 : BusSelector  OutputSignals=mdot_kgps
  Bus Selector3 : BusSelector  OutputSignals=mdot_kgps
  Bus Selector4 : BusSelector  OutputSignals=H_kJpkg
  Bus Selector5 : BusSelector  OutputSignals=mdot_kgps
  Integrator : Integrator  InitialCondition=initPres
  Integrator1 : Integrator  InitialCondition=interp2(F1.T,F1.P,F1.H_pt,initTemp,initPres)
  Liquid Enthalpy/Pressure Calcs : Subsystem
  Mux : Mux  Inputs=3
  Mux1 : Mux  Inputs=3
  T (p,h) : Lookup2D  RowIndex=F1.P  ColumnIndex=F1.H  Table=F1.T_ph  SaturateOnIntegerOverflow=on  InputSameDT=on
  Flow Out : Outport
  wires:
  Bus Selector5/1 -> Mux/3  "<mdot_kgps>"
  Flow In 3/1 -> Bus Selector5/1, Bus Selector4/1
  Bus Selector4/1 -> Mux1/3  "<H_kJpkg>"
  mdot Out/1 -> Bus Creator/4, Liquid Enthalpy/Pressure Calcs/1(Mdot_Out)  "mdot_kgps"
  Bus Creator/1 -> Flow Out/1  "Outlet"
  T (p,h)/1 -> Bus Creator/2  "temp_K"
  Flow In 1/1 -> Bus Selector/1, Bus Selector2/1  "Inlet1"
  Flow In 2/1 -> Bus Selector1/1, Bus Selector3/1  "Inlet2"
  [Pfluid] -> Liquid Enthalpy/Pressure Calcs/3(Pfluid)
  [Hfluid] -> Liquid Enthalpy/Pressure Calcs/2(Hfluid)
  Liquid Enthalpy/Pressure Calcs/2(Pdot) -> Integrator/1
  Integrator/1 -> [Pfluid], T (p,h)/1, Bus Creator/3  "pres_kPa"
  Mux/1 -> Liquid Enthalpy/Pressure Calcs/4(Mdot_In)
  Integrator1/1 -> [Hfluid], Bus Creator/1, T (p,h)/2  "H_kJpkg"
  Liquid Enthalpy/Pressure Calcs/1(Hdot) -> Integrator1/1
  Mux1/1 -> Liquid Enthalpy/Pressure Calcs/5(H_In)
  Bus Selector3/1 -> Mux/2  "<mdot_kgps>"
  Bus Selector2/1 -> Mux/1  "<mdot_kgps>"
  Bus Selector1/1 -> Mux1/2  "<H_kJpkg>"
  Bus Selector/1 -> Mux1/1  "<H_kJpkg>"

== system PowerFlowLib/Energy & Power Systems/Thermal/Fuel & Oil/Fluid Pump ==
  Flow_in : Inport
  w_rpm : Inport  Port=2
  P_out : Inport  Port=3
  (1-pf)/pf : Gain  Gain=(1-pf)/pf
  2- Lookup Table3 : Lookup_n-D  BreakpointsForDimension1=F1.P  BreakpointsForDimension2=F1.T  Table=F1.H_pt  RndMeth=Simplest  InputSameDT=on
  2pi : Gain  Gain=2*pi
  2pi/60 : Gain  Gain=2*pi()/60
  Add1 : Sum
  Add2 : Sum  Inputs=-+
  Add3 : Sum  Inputs=-+
  Bus Creator : BusCreator  Inputs=4
  Bus Creator1 : BusCreator  Inputs=3
  Bus Creator2 : BusCreator  Inputs=4
  Bus Selector : BusSelector  OutputSignals=temp_K,pres_kPa
  Constant1 : Constant  Value=pump_eff
  Cp (T,P) : Lookup_n-D  BreakpointsForDimension1=F1.P  BreakpointsForDimension2=F1.T  Table=F1.Cp_pt  RndMeth=Simplest  InputSameDT=on
  Demux : Demux  Outputs=2
  Divide2 : Product  Inputs=//*
  Divide3 : Product  Inputs=**
  Divide4 : Product  Inputs=**/
  Divide5 : Product  Inputs=**
  Divide7 : Product  Inputs=*/
  Multiport Switch : MultiPortSwitch
  Mux : Mux  Inputs=2
  Mux1 : Mux  Inputs=2
  Pump Vol. FlowRate : Lookup_n-D  NumberOfTableDimensions=1  BreakpointsForDimension1=PumpProp.B737_mech_fuel1.pres  Table=PumpProp.B737_mech_fuel1.q  RndMeth=Simplest  InputSameDT=on
  Switch : Switch  Criteria=u2 > Threshold
  Switch1 : Switch  Criteria=u2 > Threshold
  W to kW : Gain  Gain=1/1000
  data_sink : PowerFlowLib/Support Functions//Tools/data_sink
  heat_switch : Gain
  "kPa " : Gain
  kPa to Pa : Gain  Gain=1000
  kPa to bar : Gain  Gain=0.01
  kPa to m : Gain  Gain=.10197/SG
  kg/s : Gain  Gain=1/3600
  m^3/min : Gain  Gain=1/60
  pwr_switch : Constant  Value=0
  rho (T,P) : Lookup_n-D  BreakpointsForDimension1=F1.P  BreakpointsForDimension2=F1.T  Table=F1.Rho_pt  RndMeth=Simplest  InputSameDT=on
  switchcase : Constant  Value=2
  zero : Constant  Value=0
  zero1 : Constant  Value=0
  Flow_Out : Outport
  Pump Power : Outport  Port=2
  wires:
  kPa to bar/1 -> Multiport Switch/4
  "kPa "/1 -> Multiport Switch/3
  Multiport Switch/1 -> Pump Vol. FlowRate/1
  switchcase/1 -> Multiport Switch/1
  Divide4/1 -> Divide5/1  "Torq_Nm"
  Pump Vol. FlowRate/1 -> m^3/min/1, Divide3/2  "m^3/hr"
  Divide3/1 -> kg/s/1  "mdot_kgphr"
  kPa to m/1 -> Multiport Switch/2  "head (m)"
  [Pout] -> Add2/2
  [mdot] -> Bus Creator/2  "mdot_kgps"
  w_rpm/1 -> 2pi/1, 2pi/60/1, Bus Creator2/4, Switch/2, Switch/3  "shaftspeed_rpm"
  Add1/1 -> Bus Creator/3, 2- Lookup Table3/2  "temp_K"
  Add2/1 -> kPa to bar/1, "kPa "/1, kPa to m/1, kPa to Pa/1  "delta P"
  Bus Selector/2 -> Add2/1, Cp (T,P)/1, rho (T,P)/1  "<pres_kPa>"
  Bus Selector/1 -> Cp (T,P)/2, Add1/1, rho (T,P)/2  "<temp_K>"
  rho (T,P)/1 -> Divide3/1  "rho"
  Constant1/1 -> Divide7/2
  Cp (T,P)/1 -> Divide2/2
  Divide2/1 -> heat_switch/1
  Bus Creator/1 -> Flow_Out/1
  Flow_in/1 -> Bus Selector/1
  2- Lookup Table3/1 -> Bus Creator/1  "H_kJpkg"
  P_out/1 -> [Pout], Bus Creator2/2, Bus Creator/4  "pres_kPa"
  [Pout] -> 2- Lookup Table3/1
  kg/s/1 -> Switch/1
  Switch/1 -> [mdot]
  2pi/60/1 -> Divide5/2  "shftspd_rad/s"
  Divide5/1 -> Divide7/1, Add3/1  "power need"
  kPa to Pa/1 -> Divide4/1
  m^3/min/1 -> Divide4/2
  Divide7/1 -> Add3/2, Mux/1, Mux1/2  "Pump_Pwr (W)"
  2pi/1 -> Divide4/3
  Add3/1 -> W to kW/1  "heat_W"
  Demux/1 -> Bus Creator1/1  "mech_pwr_W"
  Bus Creator1/1 -> Bus Creator2/3, Pump Power/1  "Pump Pwr"
  Demux/2 -> Bus Creator1/2, (1-pf)/pf/1  "real_pwr_W"
  (1-pf)/pf/1 -> Bus Creator1/3  "react_pwr_VAr"
  Switch1/1 -> Demux/1
  pwr_switch/1 -> Switch1/2
  Mux/1 -> Switch1/1
  zero/1 -> Mux/2
  W to kW/1 -> Divide2/3
  zero1/1 -> Mux1/1
  Mux1/1 -> Switch1/3
  heat_switch/1 -> Add1/2
  Bus Creator2/1 -> data_sink/1
  [mdot] -> Bus Creator2/1  "mdot_kgps"
  [mdot] -> Divide2/1
